simulink model "AutoPID_FOC_Model_Current"  (R2022b)
settings: Solver=ode15s  StartTime=0.0  StopTime=10  MaxStep=1e-5  RelTol=1e-4
undefined symbols (not defined in the file): angle_D, angle_I, angle_P, J, kc, LPF_I, LPF_pos, LPF_speed, mode_calibration, mode_error, p, PID_angle_limit, PID_curr_D, PID_curr_I, PID_curr_limit, PID_curr_P, PID_vel_D, PID_vel_I, PID_vel_limit, PID_vel_P, step_final_angle, step_final_Iq, step_final_speed, Ts_control
libraries: fl_lib x9, nesl_utility x8, slpidlib x4, mcbcontrolslib x4, eeGeneralControl x4, ee_lib x1
settings Model: Creator=ngryaznov  LastModifiedBy=grani
settings DataIOCC: SaveOutput=off  SignalLogging=off  SaveTime=off

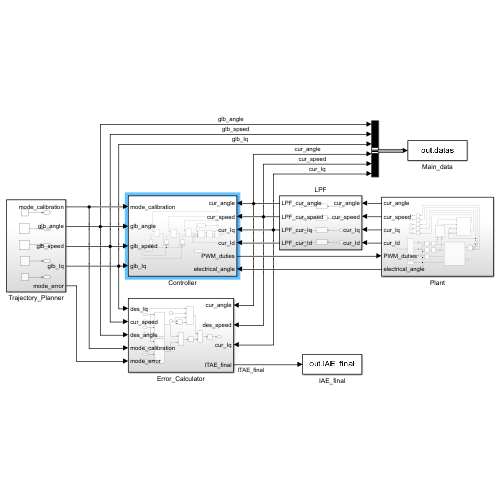
[thumbnail: Simulink's stored preview of the top-level diagram]
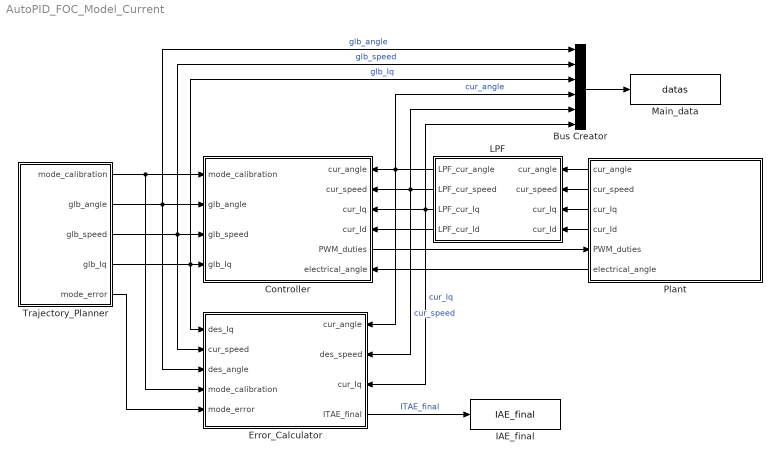
== system AutoPID_FOC_Model_Current ==
  Bus Creator : BusCreator  Inputs=6
  Controller : Subsystem
      settings: PortSchema="{\"entries\":[{\"content\":{\"sides\":[{\"content\":{\"connectorIds\":[\"In1\",\"In2\",\"In3\",\"In4\"]},\"type\":\"ConnectorPlacement.EquallySpacedRectSide\",\"uuid\":\"89a3a5e6-3177-49fe-b3a4-1a83cd7d195a\"},{\"content\":{\"connectorIds\":[\"In5\",\"In6\",\"In7\",\"In8\",\"Out1\",\"In9\"],\"side\":\"RIGHT\"},\"type\":\"ConnectorPlacement.EquallySpacedRectSide\",\"uuid\":\"705ac76c-d782-4ba6-9cf9-744d3618a946\"},{\"content\":{\"connectorIds\":[],\"side\":\"TOP\"},\"type\":\"ConnectorPlacement.EquallySpacedRectSide\",\"uuid\":\"48a18d44-c08a-4715-b03f-1a30b6a18362\"}]},\"type\":\"ConnectorPlacement.EquallySpacedConnector\",\"uuid\":\"6ebf2611-a894-48ff-b71c-8bd2ef5d571e\"}],\"packageUris\":[\"http://schema.mathworks.com/mf0/Connector/R2020b\"],\"version\":\"1.0\"}"
  Error_Calculator : Subsystem
      settings: PortSchema="{\"entries\":[{\"content\":{\"sides\":[{\"content\":{\"connectorIds\":[\"In1\",\"In2\",\"In3\",\"In4\",\"In5\"]},\"type\":\"ConnectorPlacement.EquallySpacedRectSide\",\"uuid\":\"157dec37-425b-4886-9efb-342332a52f07\"},{\"content\":{\"connectorIds\":[\"In6\",\"In7\",\"In8\",\"Out1\"],\"side\":\"RIGHT\"},\"type\":\"ConnectorPlacement.EquallySpacedRectSide\",\"uuid\":\"ea03278d-78b9-4922-b9a2-7c3b1b772f8a\"},{\"content\":{\"connectorIds\":[],\"side\":\"TOP\"},\"type\":\"ConnectorPlacement.EquallySpacedRectSide\",\"uuid\":\"f7ebc11e-576e-458d-9efe-cd47e37c6257\"}]},\"type\":\"ConnectorPlacement.EquallySpacedConnector\",\"uuid\":\"9f82fc76-bcc9-48a0-b58b-939d11dbc3f6\"}],\"packageUris\":[\"http://schema.mathworks.com/mf0/Connector/R2020b\"],\"version\":\"1.0\"}"
  IAE_final : ToWorkspace  VariableName=IAE_final  SaveFormat=Timeseries  SampleTime=-1
  LPF : Subsystem
  Main_data : ToWorkspace  VariableName=datas  SaveFormat=Timeseries  SampleTime=-1
      settings: Decimation=2
  Plant : Subsystem
      settings: PortSchema="{\"entries\":[{\"content\":{\"sides\":[{\"content\":{\"connectorIds\":[\"Out1\",\"Out2\",\"Out3\",\"Out4\",\"In1\",\"Out5\"]},\"type\":\"ConnectorPlacement.EquallySpacedRectSide\",\"uuid\":\"d82eb61f-bad1-4e87-a1c3-9ad51bbd32b3\"},{\"content\":{\"connectorIds\":[],\"side\":\"RIGHT\"},\"type\":\"ConnectorPlacement.EquallySpacedRectSide\",\"uuid\":\"4be4836c-1db7-414e-80a9-153beb1a5f11\"},{\"content\":{\"connectorIds\":[],\"side\":\"TOP\"},\"type\":\"ConnectorPlacement.EquallySpacedRectSide\",\"uuid\":\"ba067009-c59b-490e-8624-cf6c570793c3\"}]},\"type\":\"ConnectorPlacement.EquallySpacedConnector\",\"uuid\":\"f4db85a3-c362-4bc8-a2c5-e9bf326dd5c6\"}],\"packageUris\":[\"http://schema.mathworks.com/mf0/Connector/R2020b\"],\"version\":\"1.0\"}"
  Trajectory_Planner : Subsystem
  wires:
  Bus Creator/1 -> Main_data/1
  Controller/1(PWM_duties) -> Plant/1(PWM_duties)
  LPF/4(LPF_cur_Id) -> Controller/8(cur_Id)
  LPF/3(LPF_cur_Iq) -> Error_Calculator/8(cur_Iq), Bus Creator/6, Controller/7(cur_Iq)  "cur_Iq"
  LPF/2(LPF_cur_speed) -> Error_Calculator/7(des_speed), Bus Creator/5, Controller/6(cur_speed)  "cur_speed"
  LPF/1(LPF_cur_angle) -> Error_Calculator/6(cur_angle), Bus Creator/4, Controller/5(cur_angle)  "cur_angle"
  Trajectory_Planner/1(mode_calibration) -> Controller/1(mode_calibration), Error_Calculator/4(mode_calibration)
  Trajectory_Planner/2(glb_angle) -> Error_Calculator/3(des_angle), Bus Creator/1, Controller/2(glb_angle)  "glb_angle"
  Trajectory_Planner/3(glb_speed) -> Error_Calculator/2(cur_speed), Bus Creator/2, Controller/3(glb_speed)  "glb_speed"
  Trajectory_Planner/4(glb_Iq) -> Error_Calculator/1(des_Iq), Bus Creator/3, Controller/4(glb_Iq)  "glb_Iq"
  Trajectory_Planner/5(mode_error) -> Error_Calculator/5(mode_error)
  Error_Calculator/1(ITAE_final) -> IAE_final/1  "ITAE_final"
  Plant/1(cur_angle) -> LPF/1(cur_angle)
  Plant/2(cur_speed) -> LPF/2(cur_speed)
  Plant/3(cur_Iq) -> LPF/3(cur_Iq)
  Plant/4(cur_Id) -> LPF/4(cur_Id)
  Plant/5(electrical_angle) -> Controller/9(electrical_angle)

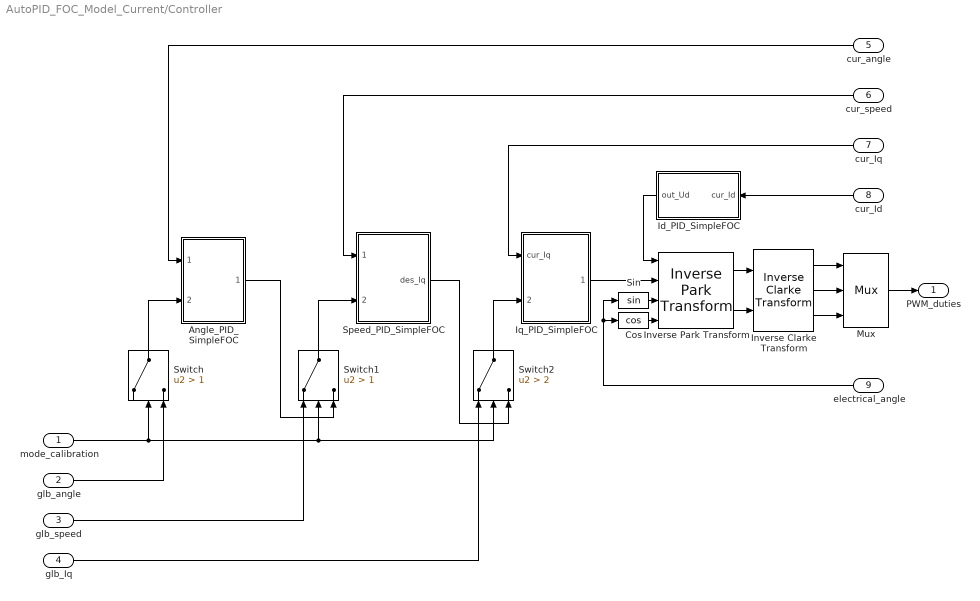
== system AutoPID_FOC_Model_Current/Controller ==
  mode_calibration : Inport
  glb_angle : Inport  Port=2
  glb_speed : Inport  Port=3
  glb_Iq : Inport  Port=4
  cur_angle : Inport  Port=5
  cur_speed : Inport  Port=6
  cur_Iq : Inport  Port=7
  cur_Id : Inport  Port=8
  electrical_angle : Inport  Port=9
  Angle_PID_SimpleFOC : Subsystem
  Cos : Trigonometry  Operator=cos
  Id_PID_SimpleFOC : Subsystem
  Inverse Clarke Transform : mcbcontrolslib/Inverse Clarke Transform
      settings: LibrarySourceBlock=mcblib/Controls/Math Transforms/Inverse Clarke Transform
  Inverse Park Transform : mcbcontrolslib/Inverse Park Transform  AxisAlignment=D-axis
      settings: LibrarySourceBlock=mcblib/Controls/Math Transforms/Inverse Park Transform
  Iq_PID_SimpleFOC : Subsystem
  Mux : Mux  Inputs=3
      settings: DisplayOption=signals
  Sin : Trigonometry
  Speed_PID_SimpleFOC : Subsystem
  Switch : Switch  Criteria=u2 > Threshold  Threshold=1  SaturateOnIntegerOverflow=off  InputSameDT=off
  Switch1 : Switch  Criteria=u2 > Threshold  Threshold=1  SaturateOnIntegerOverflow=off  InputSameDT=off
  Switch2 : Switch  Criteria=u2 > Threshold  Threshold=2  SaturateOnIntegerOverflow=off  InputSameDT=off
  PWM_duties : Outport
  wires:
  electrical_angle/1 -> Sin/1, Cos/1
  Sin/1 -> Inverse Park Transform/3
  Cos/1 -> Inverse Park Transform/4
  Inverse Park Transform/1 -> Inverse Clarke Transform/1
  Inverse Park Transform/2 -> Inverse Clarke Transform/2
  Mux/1 -> PWM_duties/1
  Inverse Clarke Transform/1 -> Mux/1
  Inverse Clarke Transform/3 -> Mux/3
  Inverse Clarke Transform/2 -> Mux/2
  cur_Id/1 -> Id_PID_SimpleFOC/1(cur_Id)
  Id_PID_SimpleFOC/1(out_Ud) -> Inverse Park Transform/1
  cur_angle/1 -> Angle_PID_SimpleFOC/1(cur_angle)
  cur_speed/1 -> Speed_PID_SimpleFOC/1(cur_speed)
  cur_Iq/1 -> Iq_PID_SimpleFOC/1(cur_Iq)
  Iq_PID_SimpleFOC/1(out_Uq) -> Inverse Park Transform/2
  mode_calibration/1 -> Switch1/2, Switch2/2, Switch/2
  glb_angle/1 -> Switch/3
  Switch2/1 -> Iq_PID_SimpleFOC/2(des_Iq)
  Switch1/1 -> Speed_PID_SimpleFOC/2(des_speed)
  Switch/1 -> Angle_PID_SimpleFOC/2(des_angle)
  Angle_PID_SimpleFOC/1(des_speed) -> Switch1/3
  glb_speed/1 -> Switch1/1
  Speed_PID_SimpleFOC/1(des_Iq) -> Switch2/3
  glb_Iq/1 -> Switch2/1

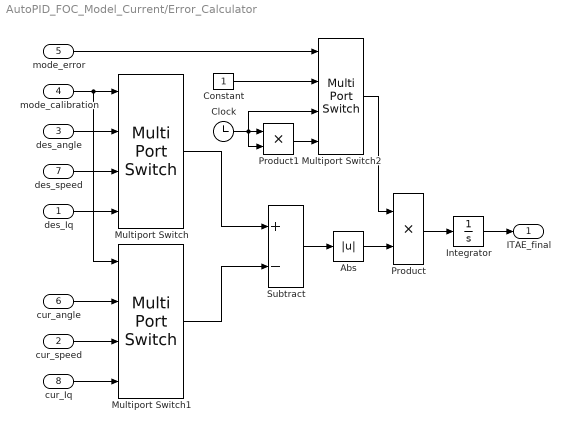
== system AutoPID_FOC_Model_Current/Error_Calculator ==
  des_Iq : Inport
  cur_speed : Inport  Port=2
  des_angle : Inport  Port=3
  mode_calibration : Inport  Port=4
  mode_error : Inport  Port=5
  cur_angle : Inport  Port=6
  des_speed : Inport  Port=7
  cur_Iq : Inport  Port=8
  Abs : Abs  SaturateOnIntegerOverflow=off
  Clock : Clock
  Constant : Constant
  Integrator : Integrator
  Multiport Switch : MultiPortSwitch  SaturateOnIntegerOverflow=off  InputSameDT=off
  Multiport Switch1 : MultiPortSwitch  SaturateOnIntegerOverflow=off  InputSameDT=off
  Multiport Switch2 : MultiPortSwitch  SaturateOnIntegerOverflow=off  InputSameDT=off
  Product : Product
  Product1 : Product
  Subtract : Sum  Inputs=+-
  ITAE_final : Outport
  wires:
  Integrator/1 -> ITAE_final/1
  Subtract/1 -> Abs/1
  Abs/1 -> Product/2
  Product/1 -> Integrator/1
  des_angle/1 -> Multiport Switch/2
  des_speed/1 -> Multiport Switch/3
  des_Iq/1 -> Multiport Switch/4
  cur_angle/1 -> Multiport Switch1/2
  cur_speed/1 -> Multiport Switch1/3
  cur_Iq/1 -> Multiport Switch1/4
  mode_calibration/1 -> Multiport Switch1/1, Multiport Switch/1
  Multiport Switch/1 -> Subtract/1
  Multiport Switch1/1 -> Subtract/2
  Constant/1 -> Multiport Switch2/2
  mode_error/1 -> Multiport Switch2/1
  Product1/1 -> Multiport Switch2/4
  Clock/1 -> Multiport Switch2/3, Product1/1, Product1/2
  Multiport Switch2/1 -> Product/1

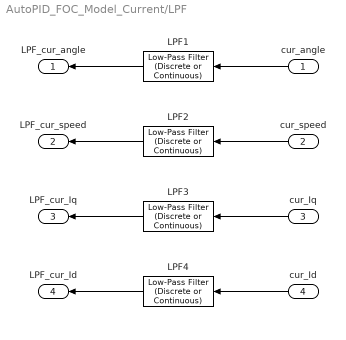
== system AutoPID_FOC_Model_Current/LPF ==
  cur_angle : Inport
  cur_speed : Inport  Port=2
  cur_Iq : Inport  Port=3
  cur_Id : Inport  Port=4
  LPF1 : eeGeneralControl/Low-Pass Filter (Discrete or Continuous)  K=1  T=LPF_pos  B=inf  A=-inf  init_option=Inherited from block input  x0=0  Ts=Ts_control
  LPF2 : eeGeneralControl/Low-Pass Filter (Discrete or Continuous)  K=1  T=LPF_speed  B=inf  A=-inf  init_option=Inherited from block input  x0=0  Ts=Ts_control
  LPF3 : eeGeneralControl/Low-Pass Filter (Discrete or Continuous)  K=1  T=LPF_I  B=inf  A=-inf  init_option=Inherited from block input  x0=0  Ts=Ts_control
  LPF4 : eeGeneralControl/Low-Pass Filter (Discrete or Continuous)  K=1  T=LPF_I  B=inf  A=-inf  init_option=Inherited from block input  x0=0  Ts=Ts_control
  LPF_cur_angle : Outport
  LPF_cur_speed : Outport  Port=2
  LPF_cur_Iq : Outport  Port=3
  LPF_cur_Id : Outport  Port=4
  wires:
  cur_angle/1 -> LPF1/1
  LPF1/1 -> LPF_cur_angle/1
  LPF2/1 -> LPF_cur_speed/1
  cur_speed/1 -> LPF2/1
  LPF3/1 -> LPF_cur_Iq/1
  cur_Iq/1 -> LPF3/1
  LPF4/1 -> LPF_cur_Id/1
  cur_Id/1 -> LPF4/1

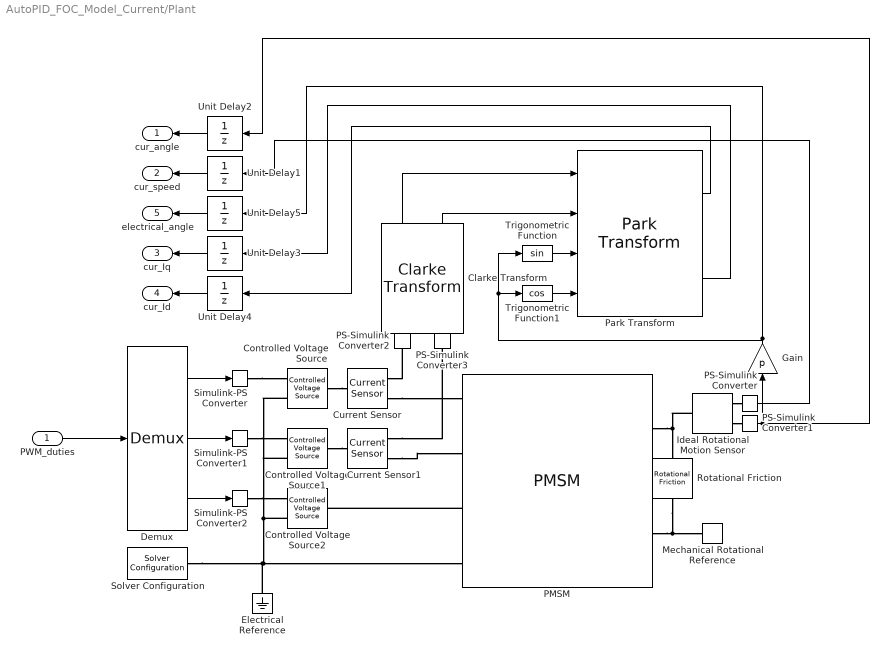
== system AutoPID_FOC_Model_Current/Plant ==
  PWM_duties : Inport
  Clarke Transform : mcbcontrolslib/Clarke Transform  VariantControl=Variant2
      settings: LibrarySourceBlock=mcblib/Controls/Math Transforms/Clarke Transform
  Controlled Voltage Source : fl_lib/Electrical/Electrical Sources/Controlled Voltage Source
  Controlled Voltage Source1 : fl_lib/Electrical/Electrical Sources/Controlled Voltage Source
  Controlled Voltage Source2 : fl_lib/Electrical/Electrical Sources/Controlled Voltage Source
  Current Sensor : fl_lib/Electrical/Electrical Sensors/Current Sensor
  Current Sensor1 : fl_lib/Electrical/Electrical Sensors/Current Sensor
  Demux : Demux  Outputs=3
      settings: DisplayOption=none
  Electrical Reference : fl_lib/Electrical/Electrical Elements/Electrical Reference
  Gain : Gain  Gain=p
  Ideal Rotational Motion Sensor : fl_lib/Mechanical/Mechanical Sensors/Ideal Rotational Motion Sensor  reference=foundation.enum.MeasurementReference.absolute  acceleration_port=false  velocity_port=true  position_port=true  wrap_angle=false  offset=0 rad
      settings: InternalSimscapePortConfiguration="{\"Bottom\":[],\"Left\":[{\"id\":\"R\",\"label\":\"R\",\"type\":\"foundation.mechanical.rotational.rotational\"}],\"Right\":[{\"id\":\"W\",\"label\":\"W\",\"type\":\"output\"},{\"id\":\"A\",\"label\":\"A\",\"type\":\"output\"}],\"Top\":[]}"
  Mechanical Rotational Reference : fl_lib/Mechanical/Rotational Elements/Mechanical Rotational Reference
  PMSM : ee_lib/Electromechanical/Permanent Magnet/PMSM  port_option=ee.enum.threePhasePort.expanded  winding_type=ee.enum.statorconnection.wye  machine_param=ee.enum.pmsm.parameterization.constant  nPolePairs=p  pmflux_param=ee.enum.pmflux.fluxlinkage  pm_flux_linkage=lambda_pm Wb  torque_constant=0.18 N*m/A  back_emf_constant=0.18 V*s/rad  stator_param=ee.enum.statorparam.LdLqL0  Ld=Ld H  Lq=Lq H  idVec=[-200, 0, 200] A  iqVec=[-200, 0, 200] A  LdMatrix=0.0002 * ones(3, 3) H  LqMatrix=0.0002 * ones(3, 3) H  PmMatrix=0.1 * ones(3, 3) Wb  ktMatrix=0.18 * ones(3, 3) N*m/A  keMatrix=0.18 * ones(3, 3) V*s/rad  L0=Ld H  Ls=0.0002 H  Lm=-0.00002 H  Ms=0.00002 H  Rs=Rs Ohm  zero_sequence=ee.enum.park.zerosequence.include  axes_param=ee.enum.rotorangle.daxis  loss_param=ee.enum.ironloss.none  losses_oc=[0, 0, 0] W  losses_sc=[0, 0, 0] W  f_losses=60 Hz  Isc_losses=95 A  J=J kg*m^2  lam=B N*m*s/rad  i_d_specify=off  i_d_priority=None  i_d=0 A  i_d_nominal_specify=off  i_d_nominal_unit=A  i_d_nominal_value=1  i_q_specify=off  i_q_priority=None  i_q=0 A  i_q_nominal_specify=off  i_q_nominal_unit=A  i_q_nominal_value=1  torque_specify=off  torque_priority=None  torque=0 N*m  torque_nominal_specify=off  torque_nominal_unit=N*m  torque_nominal_value=1  angular_velocity_specify=off  angular_velocity_priority=High  angular_velocity=0 rpm  angular_velocity_nominal_specify=off  angular_velocity_nominal_unit=rpm  angular_velocity_nominal_value=1  angular_position_specify=off  angular_position_priority=High  angular_position=0 deg  angular_position_nominal_specify=off  angular_position_nominal_unit=deg  angular_position_nominal_value=1  alpha=3.93e-3 1/K  alpha_flux=-0.001 1/K  Tmeas=298.15 K  stator_thermal_mass=100 J/K  rotor_thermal_mass=200 J/K  Rm_percent_rotor=90  Rd_percent_rotor=30  temperatureA_specify=off  temperatureA_priority=High  temperatureA=25 degC  temperatureA_nominal_specify=off  temperatureA_nominal_unit=degC  temperatureA_nominal_value=1  temperatureB_specify=off  temperatureB_priority=High  temperatureB=25 degC  temperatureB_nominal_specify=off  temperatureB_nominal_unit=degC  temperatureB_nominal_value=1  temperatureC_specify=off  temperatureC_priority=High  temperatureC=25 degC  temperatureC_nominal_specify=off  temperatureC_nominal_unit=degC  temperatureC_nominal_value=1  temperatureR_specify=off  temperatureR_priority=High  temperatureR=25 degC  temperatureR_nominal_specify=off  temperatureR_nominal_unit=degC  temperatureR_nominal_value=1
      settings: InternalSimscapePortConfiguration="{\"Bottom\":[],\"Left\":[{\"id\":\"a\",\"label\":\"a\",\"type\":\"foundation.electrical.electrical\"},{\"id\":\"b\",\"label\":\"b\",\"type\":\"foundation.electrical.electrical\"},{\"id\":\"c\",\"label\":\"c\",\"type\":\"foundation.electrical.electrical\"},{\"id\":\"n\",\"label\":\"n\",\"type\":\"foundation.electrical.electrical\"}],\"Right\":[{\"id\":\"R\",\"label\":\"R\",\"type\":\"foundation.mechanical.rotational.rotational\"},{\"id\":\"C\",\"label\":\"C\",\"type\":\"foundation.mechanical.rotational.rotational\"}],\"Top\":[]}"
  PS-Simulink Converter{,1..3} (4 alike) : nesl_utility/PS-Simulink Converter  PhysicalDomain=network_engine_domain  SubClassName=ps_output  LeftPortType=input  RightPortType=output  PseudoPeriodic=off  Frequencies=[]  VectorFormat=inherit  Unit=inherit  AffineConversion=off
  Park Transform : mcbcontrolslib/Park Transform  AxisAlignment=D-axis
      settings: LibrarySourceBlock=mcblib/Controls/Math Transforms/Park Transform
  Rotational Friction : fl_lib/Mechanical/Rotational Elements/Rotational Friction  brkwy_trq=0.0005 N*m  brkwy_vel=0.01 rad/s  Col_trq=0.0002 N*m  visc_coef=0 N*m*s/rad  w_specify=off  w_priority=None  w=0 rad/s  w_nominal_specify=off  w_nominal_unit=rad/s  w_nominal_value=1  t_specify=off  t_priority=None  t=0 N*m  t_nominal_specify=off  t_nominal_unit=N*m  t_nominal_value=1
  Simulink-PS Converter : nesl_utility/Simulink-PS Converter  PhysicalDomain=network_engine_domain  SubClassName=ps_input  LeftPortType=input  RightPortType=output  PseudoPeriodic=off  Frequencies=[]  NoiseDistribution=none  NoiseParameters=[]  Unit=1  AffineConversion=off  FilteringAndDerivatives=provide  SimscapeFilterOrder=1  InputFilterTimeConstant=0.001  UdotUserProvided=0
  Simulink-PS Converter1 : nesl_utility/Simulink-PS Converter  PhysicalDomain=network_engine_domain  SubClassName=ps_input  LeftPortType=input  RightPortType=output  PseudoPeriodic=off  Frequencies=[]  NoiseDistribution=none  NoiseParameters=[]  Unit=1  AffineConversion=off  FilteringAndDerivatives=provide  SimscapeFilterOrder=1  InputFilterTimeConstant=0.001  UdotUserProvided=0
  Simulink-PS Converter2 : nesl_utility/Simulink-PS Converter  PhysicalDomain=network_engine_domain  SubClassName=ps_input  LeftPortType=input  RightPortType=output  PseudoPeriodic=off  Frequencies=[]  NoiseDistribution=none  NoiseParameters=[]  Unit=1  AffineConversion=off  FilteringAndDerivatives=provide  SimscapeFilterOrder=1  InputFilterTimeConstant=0.001  UdotUserProvided=0
  Solver Configuration : nesl_utility/Solver Configuration  PhysicalDomain=network_engine_domain  SubClassName=solver  LeftPortType=input  RightPortType=generic  Tones=[]  Harmonics=[]  SimulateNoise=off  Profile=off  UseLocalSampling=off  EnableSwitchedLinearOptims=on  FrequencyDomain=off  UseCCode=off  RelTol=0.001  AbsTol=0.001  MinStep=1e-09  ToWorkspace=off  RevertToSquareIcSolve=off  NumHomotopyIterations=100  PhasorMode=off  PhasorModeNumHarmonics=1  ConsistencySolver=NEWTON_XTOL_AFTER_FTOL  IndexReductionMethod=DerivativeReplacement  DoDC=off  ResidualTolerance=1e-09  ConsistencyTolSource=GLOBAL  ConsistencyAbsTol=0.001  ConsistencyRelTol=0.001  ConsistencyTolFactor=0.001  UseLocalSolver=on  LocalSolverChoice=NE_BACKWARD_EULER_ADVANCER  ResolveIndetEquations=on  FunctionEvalNumThread=1  LocalSolverSampleTime=0.001  DoFixedCost=on  MaxNonlinIter=3  MaxModeIter=2  ComputeImpulses=off  ImpulseIterations=2  LinearAlgebra=auto  LinearAlgebraNumThread=0  EquationFormulation=NE_TIME_EF  DelaysMemoryBudget=1024  AutomaticFiltering=on  FilteringTimeConstant=0.001  PartitionStorageMethod=AS_NEEDED  PartitionMemoryBudget=1024  PartitionMethod=ROBUST
  Trigonometric Function : Trigonometry
  Trigonometric Function1 : Trigonometry  Operator=cos
  Unit Delay{1..5} (5 alike) : UnitDelay  SampleTime=Ts_control  HasFrameUpgradeWarning=on
  cur_angle : Outport
  cur_speed : Outport  Port=2
  cur_Iq : Outport  Port=3
  cur_Id : Outport  Port=4
  electrical_angle : Outport  Port=5
  wires:
  PS-Simulink Converter/1 -> Unit Delay1/1
  PS-Simulink Converter1/1 -> Gain/1, Unit Delay2/1
  PS-Simulink Converter2/1 -> Clarke Transform/1
  PS-Simulink Converter3/1 -> Clarke Transform/2
  Clarke Transform/1 -> Park Transform/1
  Clarke Transform/2 -> Park Transform/2
  Trigonometric Function1/1 -> Park Transform/4
  Trigonometric Function/1 -> Park Transform/3
  PWM_duties/1 -> Demux/1
  Gain/1 -> Trigonometric Function/1, Trigonometric Function1/1, Unit Delay5/1
  Demux/1 -> Simulink-PS Converter/1
  Demux/2 -> Simulink-PS Converter1/1
  Demux/3 -> Simulink-PS Converter2/1
  Unit Delay1/1 -> cur_speed/1
  Unit Delay2/1 -> cur_angle/1
  Unit Delay3/1 -> cur_Iq/1
  Unit Delay4/1 -> cur_Id/1
  Unit Delay5/1 -> electrical_angle/1
  Park Transform/1 -> Unit Delay4/1
  Park Transform/2 -> Unit Delay3/1
  connections:
  Simulink-PS Converter/RConn1 -- Controlled Voltage Source/RConn1
  Simulink-PS Converter1/RConn1 -- Controlled Voltage Source1/RConn1
  Simulink-PS Converter2/RConn1 -- Controlled Voltage Source2/RConn1
  Controlled Voltage Source/LConn1 -- Current Sensor/LConn1
  Controlled Voltage Source1/LConn1 -- Current Sensor1/LConn1
  PMSM/LConn3 -- Controlled Voltage Source2/LConn1
  Current Sensor/RConn2 -- PMSM/LConn1
  Current Sensor1/RConn2 -- PMSM/LConn2
  Electrical Reference/LConn1 -- PMSM/LConn4 -- Controlled Voltage Source/RConn2 -- Controlled Voltage Source1/RConn2 -- Controlled Voltage Source2/RConn2 -- Solver Configuration/RConn1
  PMSM/RConn1 -- Rotational Friction/LConn1 -- Ideal Rotational Motion Sensor/LConn1
  Current Sensor/RConn1 -- PS-Simulink Converter2/LConn1
  Current Sensor1/RConn1 -- PS-Simulink Converter3/LConn1
  Ideal Rotational Motion Sensor/RConn2 -- PS-Simulink Converter1/LConn1
  Ideal Rotational Motion Sensor/RConn1 -- PS-Simulink Converter/LConn1
  PMSM/RConn2 -- Rotational Friction/RConn1 -- Mechanical Rotational Reference/LConn1

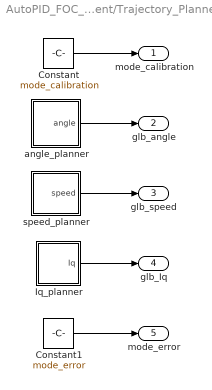
== system AutoPID_FOC_Model_Current/Trajectory_Planner ==
  Constant : Constant  Value=mode_calibration
  Constant1 : Constant  Value=mode_error
  Iq_planner : Subsystem
  angle_planner : Subsystem
  speed_planner : Subsystem
  mode_calibration : Outport
  glb_angle : Outport  Port=2
  glb_speed : Outport  Port=3
  glb_Iq : Outport  Port=4
  mode_error : Outport  Port=5
  wires:
  Constant/1 -> mode_calibration/1
  angle_planner/1(angle) -> glb_angle/1
  speed_planner/1(speed) -> glb_speed/1
  Iq_planner/1(Iq) -> glb_Iq/1
  Constant1/1 -> mode_error/1

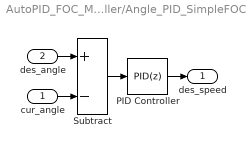
== system AutoPID_FOC_Model_Current/Controller/Angle_PID_SimpleFOC ==
  cur_angle : Inport
  des_angle : Inport  Port=2
  PID Controller : slpidlib/PID Controller  Controller=PID  Form=Parallel  TimeDomain=Discrete-time  UseExternalTs=off  SampleTime=Ts_control  IntegratorMethod=Trapezoidal  FilterMethod=Trapezoidal  ControllerParametersSource=internal  P=angle_P  I=angle_I  UseKiTs=off  D=angle_D  N=100  UseFilter=on  TunerSelectOption=Transfer Function Based (PID Tuner App)  InitialConditionSource=internal  InitialConditionForIntegrator=0  InitialConditionForFilter=0  DifferentiatorICPrevScaledInput=0  ExternalReset=none  TrackingMode=off  Kt=1  LimitOutput=on  SatLimitsSource=internal  UpperSaturationLimit=PID_angle_limit  LowerSaturationLimit=-PID_angle_limit  LinearizeAsGain=off  AntiWindupMode=none  Kb=kc  LimitIntegrator=off  UpperIntegratorSaturationLimit=inf  LowerIntegratorSaturationLimit=-inf  POutMin=[]  POutMax=[]  IOutMin=[]  IOutMax=[]  DOutMin=[]  DOutMax=[]  NOutMin=[]  NOutMax=[]  SumOutMin=[]  SumOutMax=[]  SaturationOutMin=[]  SaturationOutMax=[]  PParamMin=[]  PParamMax=[]  IParamMin=[]  IParamMax=[]  DParamMin=[]  DParamMax=[]  NParamMin=[]  NParamMax=[]  KbParamMin=[]  KbParamMax=[]  KtParamMin=[]  KtParamMax=[]  KbOutMin=[]  KbOutMax=[]  KtOutMin=[]  KtOutMax=[]  IntegratorOutMin=[]  IntegratorOutMax=[]  FilterOutMin=[]  FilterOutMax=[]  SumI1OutMin=[]  SumI1OutMax=[]  SumI2OutMin=[]  SumI2OutMax=[]  SumI3OutMin=[]  SumI3OutMax=[]  SumI4OutMin=[]  SumI4OutMax=[]  SumDOutMin=[]  SumDOutMax=[]  DifferentiatorOutMin=[]  DifferentiatorOutMax=[]  FilterDiffOutCoefMin=[]  FilterDiffOutCoefMax=[]  ReciprocalOutMin=[]  ReciprocalOutMax=[]  SumDenOutMin=[]  SumDenOutMax=[]  SumNumOutMin=[]  SumNumOutMax=[]  DivideOutMin=[]  DivideOutMax=[]  UdiffTsProdOutMin=[]  UdiffTsProdOutMax=[]  NTsProdOutMin=[]  NTsProdOutMax=[]  UintegralTsProdOutMin=[]  UintegralTsProdOutMax=[]  UngainTsProdOutMin=[]  UngainTsProdOutMax=[]  ClampingZeroOutDataTypeStr=Inherit: Inherit via back propagation  ClampingZeroOutMin=[]  ClampingZeroOutMax=[]  FilterDenConstantOutDataTypeStr=Inherit: Inherit via back propagation  FilterDenConstantOutMin=[]  FilterDenConstantOutMax=[]  PCopyOutDataTypeStr=Inherit: Inherit via back propagation  PCopyOutMin=[]  PCopyOutMax=[]  NCopyOutDataTypeStr=Inherit: Inherit via back propagation  NCopyOutMin=[]  NCopyOutMax=[]  IntegratorContinuousStateAttributes=''  IntegratorStateMustResolveToSignalObject=off  IntegratorRTWStateStorageClass=Auto  FilterContinuousStateAttributes=''  FilterStateMustResolveToSignalObject=off  FilterRTWStateStorageClass=Auto  ParallelPVariant=InternalParameters  IdealPVariant=Disabled  IVariant=InternalParameters  DVariant=InternalParameters  IntegratorVariant=Discrete  SatVariant=Enabled  AWVariant=Passthrough  PCopyVariant=Disabled  TRVariant=Disabled  FdbkBlocksVariant=Forward  IdealPFdbkVariant=Disabled  SatFdbkVariant=Disabled  DerivativeFilterVariant=TrapezoidalFilter  NVariant=InternalParameters  NCopyVariant=InternalParameters  FilterICVariant=InternalICsFilter  IntegratorICVariant=InternalICs  ExternalResetVariant=Disabled  TRSumVariant=Passthrough  SumFdbkVariant=Disabled  SumVariant=Sum_PID  TsampFilterVariant=InternalTs  TsampNgainVariant=Passthrough  TsampIntegralVariant=Passthrough  ExternalSaturationOutDataTypeStr=Inherit: Same as second input
  Subtract : Sum  Inputs=+-
  des_speed : Outport
  wires:
  des_angle/1 -> Subtract/1
  cur_angle/1 -> Subtract/2
  Subtract/1 -> PID Controller/1
  PID Controller/1 -> des_speed/1

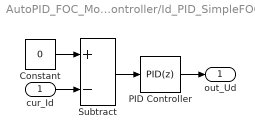
== system AutoPID_FOC_Model_Current/Controller/Id_PID_SimpleFOC ==
  cur_Id : Inport
  Constant : Constant  Value=0
  PID Controller : slpidlib/PID Controller  Controller=PID  Form=Parallel  TimeDomain=Discrete-time  UseExternalTs=off  SampleTime=Ts_control  IntegratorMethod=Trapezoidal  FilterMethod=Trapezoidal  ControllerParametersSource=internal  P=PID_curr_P  I=PID_curr_I  UseKiTs=off  D=PID_curr_D  N=100  UseFilter=on  TunerSelectOption=Transfer Function Based (PID Tuner App)  InitialConditionSource=internal  InitialConditionForIntegrator=0  InitialConditionForFilter=0  DifferentiatorICPrevScaledInput=0  ExternalReset=none  TrackingMode=off  Kt=1  LimitOutput=on  SatLimitsSource=internal  UpperSaturationLimit=PID_curr_limit  LowerSaturationLimit=-PID_curr_limit  LinearizeAsGain=off  AntiWindupMode=back-calculation  Kb=kc  LimitIntegrator=off  UpperIntegratorSaturationLimit=inf  LowerIntegratorSaturationLimit=-inf  POutMin=[]  POutMax=[]  IOutMin=[]  IOutMax=[]  DOutMin=[]  DOutMax=[]  NOutMin=[]  NOutMax=[]  SumOutMin=[]  SumOutMax=[]  SaturationOutMin=[]  SaturationOutMax=[]  PParamMin=[]  PParamMax=[]  IParamMin=[]  IParamMax=[]  DParamMin=[]  DParamMax=[]  NParamMin=[]  NParamMax=[]  KbParamMin=[]  KbParamMax=[]  KtParamMin=[]  KtParamMax=[]  KbOutMin=[]  KbOutMax=[]  KtOutMin=[]  KtOutMax=[]  IntegratorOutMin=[]  IntegratorOutMax=[]  FilterOutMin=[]  FilterOutMax=[]  SumI1OutMin=[]  SumI1OutMax=[]  SumI2OutMin=[]  SumI2OutMax=[]  SumI3OutMin=[]  SumI3OutMax=[]  SumI4OutMin=[]  SumI4OutMax=[]  SumDOutMin=[]  SumDOutMax=[]  DifferentiatorOutMin=[]  DifferentiatorOutMax=[]  FilterDiffOutCoefMin=[]  FilterDiffOutCoefMax=[]  ReciprocalOutMin=[]  ReciprocalOutMax=[]  SumDenOutMin=[]  SumDenOutMax=[]  SumNumOutMin=[]  SumNumOutMax=[]  DivideOutMin=[]  DivideOutMax=[]  UdiffTsProdOutMin=[]  UdiffTsProdOutMax=[]  NTsProdOutMin=[]  NTsProdOutMax=[]  UintegralTsProdOutMin=[]  UintegralTsProdOutMax=[]  UngainTsProdOutMin=[]  UngainTsProdOutMax=[]  ClampingZeroOutDataTypeStr=Inherit: Inherit via back propagation  ClampingZeroOutMin=[]  ClampingZeroOutMax=[]  FilterDenConstantOutDataTypeStr=Inherit: Inherit via back propagation  FilterDenConstantOutMin=[]  FilterDenConstantOutMax=[]  PCopyOutDataTypeStr=Inherit: Inherit via back propagation  PCopyOutMin=[]  PCopyOutMax=[]  NCopyOutDataTypeStr=Inherit: Inherit via back propagation  NCopyOutMin=[]  NCopyOutMax=[]  IntegratorContinuousStateAttributes=''  IntegratorStateMustResolveToSignalObject=off  IntegratorRTWStateStorageClass=Auto  FilterContinuousStateAttributes=''  FilterStateMustResolveToSignalObject=off  FilterRTWStateStorageClass=Auto  ParallelPVariant=InternalParameters  IdealPVariant=Disabled  IVariant=InternalParameters  DVariant=InternalParameters  IntegratorVariant=Discrete  SatVariant=Enabled  AWVariant=BackCalculation  PCopyVariant=Disabled  TRVariant=Disabled  FdbkBlocksVariant=Feedback  IdealPFdbkVariant=Passthrough  SatFdbkVariant=Enabled  DerivativeFilterVariant=TrapezoidalFilter  NVariant=InternalParameters  NCopyVariant=InternalParameters  FilterICVariant=InternalICsFilter  IntegratorICVariant=InternalICs  ExternalResetVariant=Disabled  TRSumVariant=Passthrough  SumFdbkVariant=Enabled  SumVariant=Sum_PID  TsampFilterVariant=InternalTs  TsampNgainVariant=Passthrough  TsampIntegralVariant=Passthrough  ExternalSaturationOutDataTypeStr=Inherit: Same as second input
  Subtract : Sum  Inputs=+-
  out_Ud : Outport
  wires:
  cur_Id/1 -> Subtract/2
  Subtract/1 -> PID Controller/1
  PID Controller/1 -> out_Ud/1
  Constant/1 -> Subtract/1

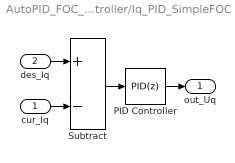
== system AutoPID_FOC_Model_Current/Controller/Iq_PID_SimpleFOC ==
  cur_Iq : Inport
  des_Iq : Inport  Port=2
  PID Controller : slpidlib/PID Controller  Controller=PID  Form=Parallel  TimeDomain=Discrete-time  UseExternalTs=off  SampleTime=Ts_control  IntegratorMethod=Trapezoidal  FilterMethod=Trapezoidal  ControllerParametersSource=internal  P=PID_curr_P  I=PID_curr_I  UseKiTs=off  D=PID_curr_D  N=100  UseFilter=on  TunerSelectOption=Transfer Function Based (PID Tuner App)  InitialConditionSource=internal  InitialConditionForIntegrator=0  InitialConditionForFilter=0  DifferentiatorICPrevScaledInput=0  ExternalReset=none  TrackingMode=off  Kt=1  LimitOutput=on  SatLimitsSource=internal  UpperSaturationLimit=PID_curr_limit  LowerSaturationLimit=-PID_curr_limit  LinearizeAsGain=off  AntiWindupMode=back-calculation  Kb=kc  LimitIntegrator=off  UpperIntegratorSaturationLimit=inf  LowerIntegratorSaturationLimit=-inf  POutMin=[]  POutMax=[]  IOutMin=[]  IOutMax=[]  DOutMin=[]  DOutMax=[]  NOutMin=[]  NOutMax=[]  SumOutMin=[]  SumOutMax=[]  SaturationOutMin=[]  SaturationOutMax=[]  PParamMin=[]  PParamMax=[]  IParamMin=[]  IParamMax=[]  DParamMin=[]  DParamMax=[]  NParamMin=[]  NParamMax=[]  KbParamMin=[]  KbParamMax=[]  KtParamMin=[]  KtParamMax=[]  KbOutMin=[]  KbOutMax=[]  KtOutMin=[]  KtOutMax=[]  IntegratorOutMin=[]  IntegratorOutMax=[]  FilterOutMin=[]  FilterOutMax=[]  SumI1OutMin=[]  SumI1OutMax=[]  SumI2OutMin=[]  SumI2OutMax=[]  SumI3OutMin=[]  SumI3OutMax=[]  SumI4OutMin=[]  SumI4OutMax=[]  SumDOutMin=[]  SumDOutMax=[]  DifferentiatorOutMin=[]  DifferentiatorOutMax=[]  FilterDiffOutCoefMin=[]  FilterDiffOutCoefMax=[]  ReciprocalOutMin=[]  ReciprocalOutMax=[]  SumDenOutMin=[]  SumDenOutMax=[]  SumNumOutMin=[]  SumNumOutMax=[]  DivideOutMin=[]  DivideOutMax=[]  UdiffTsProdOutMin=[]  UdiffTsProdOutMax=[]  NTsProdOutMin=[]  NTsProdOutMax=[]  UintegralTsProdOutMin=[]  UintegralTsProdOutMax=[]  UngainTsProdOutMin=[]  UngainTsProdOutMax=[]  ClampingZeroOutDataTypeStr=Inherit: Inherit via back propagation  ClampingZeroOutMin=[]  ClampingZeroOutMax=[]  FilterDenConstantOutDataTypeStr=Inherit: Inherit via back propagation  FilterDenConstantOutMin=[]  FilterDenConstantOutMax=[]  PCopyOutDataTypeStr=Inherit: Inherit via back propagation  PCopyOutMin=[]  PCopyOutMax=[]  NCopyOutDataTypeStr=Inherit: Inherit via back propagation  NCopyOutMin=[]  NCopyOutMax=[]  IntegratorContinuousStateAttributes=''  IntegratorStateMustResolveToSignalObject=off  IntegratorRTWStateStorageClass=Auto  FilterContinuousStateAttributes=''  FilterStateMustResolveToSignalObject=off  FilterRTWStateStorageClass=Auto  ParallelPVariant=InternalParameters  IdealPVariant=Disabled  IVariant=InternalParameters  DVariant=InternalParameters  IntegratorVariant=Discrete  SatVariant=Enabled  AWVariant=BackCalculation  PCopyVariant=Disabled  TRVariant=Disabled  FdbkBlocksVariant=Feedback  IdealPFdbkVariant=Passthrough  SatFdbkVariant=Enabled  DerivativeFilterVariant=TrapezoidalFilter  NVariant=InternalParameters  NCopyVariant=InternalParameters  FilterICVariant=InternalICsFilter  IntegratorICVariant=InternalICs  ExternalResetVariant=Disabled  TRSumVariant=Passthrough  SumFdbkVariant=Enabled  SumVariant=Sum_PID  TsampFilterVariant=InternalTs  TsampNgainVariant=Passthrough  TsampIntegralVariant=Passthrough  ExternalSaturationOutDataTypeStr=Inherit: Same as second input
  Subtract : Sum  Inputs=+-
  out_Uq : Outport
  wires:
  PID Controller/1 -> out_Uq/1
  des_Iq/1 -> Subtract/1
  cur_Iq/1 -> Subtract/2
  Subtract/1 -> PID Controller/1

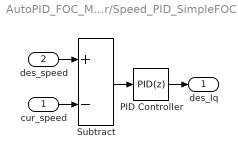
== system AutoPID_FOC_Model_Current/Controller/Speed_PID_SimpleFOC ==
  cur_speed : Inport
  des_speed : Inport  Port=2
  PID Controller : slpidlib/PID Controller  Controller=PID  Form=Parallel  TimeDomain=Discrete-time  UseExternalTs=off  SampleTime=Ts_control  IntegratorMethod=Trapezoidal  FilterMethod=Trapezoidal  ControllerParametersSource=internal  P=PID_vel_P  I=PID_vel_I  UseKiTs=off  D=PID_vel_D  N=100  UseFilter=on  TunerSelectOption=Transfer Function Based (PID Tuner App)  InitialConditionSource=internal  InitialConditionForIntegrator=0  InitialConditionForFilter=0  DifferentiatorICPrevScaledInput=0  ExternalReset=none  TrackingMode=off  Kt=1  LimitOutput=on  SatLimitsSource=internal  UpperSaturationLimit=PID_vel_limit  LowerSaturationLimit=-PID_vel_limit  LinearizeAsGain=off  AntiWindupMode=back-calculation  Kb=kc  LimitIntegrator=off  UpperIntegratorSaturationLimit=inf  LowerIntegratorSaturationLimit=-inf  POutMin=[]  POutMax=[]  IOutMin=[]  IOutMax=[]  DOutMin=[]  DOutMax=[]  NOutMin=[]  NOutMax=[]  SumOutMin=[]  SumOutMax=[]  SaturationOutMin=[]  SaturationOutMax=[]  PParamMin=[]  PParamMax=[]  IParamMin=[]  IParamMax=[]  DParamMin=[]  DParamMax=[]  NParamMin=[]  NParamMax=[]  KbParamMin=[]  KbParamMax=[]  KtParamMin=[]  KtParamMax=[]  KbOutMin=[]  KbOutMax=[]  KtOutMin=[]  KtOutMax=[]  IntegratorOutMin=[]  IntegratorOutMax=[]  FilterOutMin=[]  FilterOutMax=[]  SumI1OutMin=[]  SumI1OutMax=[]  SumI2OutMin=[]  SumI2OutMax=[]  SumI3OutMin=[]  SumI3OutMax=[]  SumI4OutMin=[]  SumI4OutMax=[]  SumDOutMin=[]  SumDOutMax=[]  DifferentiatorOutMin=[]  DifferentiatorOutMax=[]  FilterDiffOutCoefMin=[]  FilterDiffOutCoefMax=[]  ReciprocalOutMin=[]  ReciprocalOutMax=[]  SumDenOutMin=[]  SumDenOutMax=[]  SumNumOutMin=[]  SumNumOutMax=[]  DivideOutMin=[]  DivideOutMax=[]  UdiffTsProdOutMin=[]  UdiffTsProdOutMax=[]  NTsProdOutMin=[]  NTsProdOutMax=[]  UintegralTsProdOutMin=[]  UintegralTsProdOutMax=[]  UngainTsProdOutMin=[]  UngainTsProdOutMax=[]  ClampingZeroOutDataTypeStr=Inherit: Inherit via back propagation  ClampingZeroOutMin=[]  ClampingZeroOutMax=[]  FilterDenConstantOutDataTypeStr=Inherit: Inherit via back propagation  FilterDenConstantOutMin=[]  FilterDenConstantOutMax=[]  PCopyOutDataTypeStr=Inherit: Inherit via back propagation  PCopyOutMin=[]  PCopyOutMax=[]  NCopyOutDataTypeStr=Inherit: Inherit via back propagation  NCopyOutMin=[]  NCopyOutMax=[]  IntegratorContinuousStateAttributes=''  IntegratorStateMustResolveToSignalObject=off  IntegratorRTWStateStorageClass=Auto  FilterContinuousStateAttributes=''  FilterStateMustResolveToSignalObject=off  FilterRTWStateStorageClass=Auto  ParallelPVariant=InternalParameters  IdealPVariant=Disabled  IVariant=InternalParameters  DVariant=InternalParameters  IntegratorVariant=Discrete  SatVariant=Enabled  AWVariant=BackCalculation  PCopyVariant=Disabled  TRVariant=Disabled  FdbkBlocksVariant=Feedback  IdealPFdbkVariant=Passthrough  SatFdbkVariant=Enabled  DerivativeFilterVariant=TrapezoidalFilter  NVariant=InternalParameters  NCopyVariant=InternalParameters  FilterICVariant=InternalICsFilter  IntegratorICVariant=InternalICs  ExternalResetVariant=Disabled  TRSumVariant=Passthrough  SumFdbkVariant=Enabled  SumVariant=Sum_PID  TsampFilterVariant=InternalTs  TsampNgainVariant=Passthrough  TsampIntegralVariant=Passthrough  ExternalSaturationOutDataTypeStr=Inherit: Same as second input
  Subtract : Sum  Inputs=+-
  des_Iq : Outport
  wires:
  des_speed/1 -> Subtract/1
  cur_speed/1 -> Subtract/2
  Subtract/1 -> PID Controller/1
  PID Controller/1 -> des_Iq/1

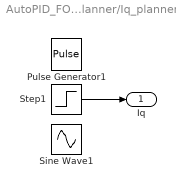
== system AutoPID_FOC_Model_Current/Trajectory_Planner/Iq_planner ==
  Pulse Generator1 : DiscretePulseGenerator  PulseType=Time based  Period=18  PulseWidth=50
  Sine Wave1 : Sin  Frequency=2*pi*0.1  SampleTime=0
  Step1 : Step  Time=0.01  After=step_final_Iq  SampleTime=Ts_control
  Iq : Outport
  wires:
  Step1/1 -> Iq/1

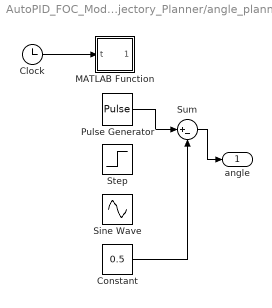
== system AutoPID_FOC_Model_Current/Trajectory_Planner/angle_planner ==
  Clock : Clock
  Constant : Constant  Value=0.5
  MATLAB Function : MATLAB Function  TreatAsAtomicUnit=on
  Pulse Generator : DiscretePulseGenerator  PulseType=Time based  Period=4  PulseWidth=50
  Sine Wave : Sin  Frequency=2*pi*0.1  SampleTime=0
  Step : Step  Time=0.01  After=step_final_angle  SampleTime=Ts_control
  Sum : Sum  Inputs=|+-
  angle : Outport
  wires:
  Clock/1 -> MATLAB Function/1(t)
  Pulse Generator/1 -> Sum/1
  Constant/1 -> Sum/2
  Sum/1 -> angle/1

== system AutoPID_FOC_Model_Current/Trajectory_Planner/speed_planner ==
  Pulse Generator2 : DiscretePulseGenerator  PulseType=Time based  Amplitude=20  Period=18  PulseWidth=50
  Sine Wave2 : Sin  Amplitude=20  Frequency=2*pi*0.2  SampleTime=0
  Step3 : Step  Time=0.01  After=step_final_speed  SampleTime=Ts_control
  speed : Outport
  wires:
  Step3/1 -> speed/1

== matlab function AutoPID_FOC_Model_Current/Trajectory_Planner/angle_planner/MATLAB Function ==
  data: t input; theta output
function theta = flyby_angle(t)
% ============================================================
%  Генератор угла цели для пролёта объекта мимо установки
%  (для блока MATLAB Function в Simulink)
%
%  Вход:  t   - время (с), t=0 соответствует позиции x = -l
%  Выход: theta - угол в радианах (всегда >= 0)
%
%  Геометрия:
%    - Установка в (0,0)
%    - Объект летит параллельно оси X на расстоянии h
%    - x(t) = -l + v*t
%    - Угол отсчитывается от направления "параллельно траектории"
%      со стороны приближения (отрицательное направление X)
%
%  После того как объект ушёл за x = +l — угол фиксируется
%  на последнем значении.
% ============================================================

    % ================== ПАРАМЕТРЫ (Измени под себя) ==================
    h = 200;      % [м]   минимальное расстояние от установки до траектории (impact parameter)
    v = 1800;     % [м/с] скорость объекта (постоянная)
    l = 2000;    % [м]   расстояние от точки минимального сближения до начала/конца участка
    % ================================================================

    % Текущая координата объекта вдоль траектории
    x = -l + v * t;

    % После прохождения точки x = +l держим последнее значение угла
    if x > l
        x = l;
    end

    % Основная формула угла
    % (pi - atan2(h, x)) даёт:
    %   - в начале (x=-l) → угол близок к 0
    %   - в момент минимального расстояния (x=0) → pi/2
    %   - в конце (x=+l) → угол близок к pi (но меньше)
    theta = pi - atan2(h, x);

end
